simulink model "rl_forced_response"  (R2014b)
settings: Solver=ode45  StartTime=0.0  StopTime=1  RelTol=1e-3
libraries: powerlib x5
settings Model: Creator=Mashkoor Ahmed  LastModifiedBy=Mashkoor Ahmed

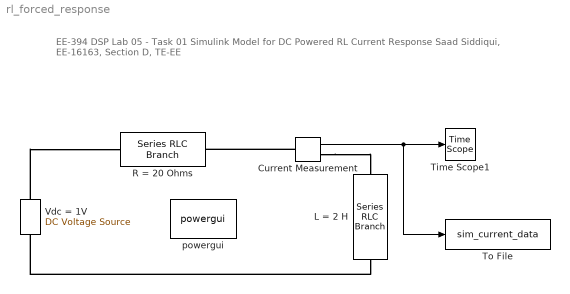
== system rl_forced_response ==
  note: EE-394 DSP Lab 05 - Task 01
      | Simulink Model for DC Powered RL Current Response
      | Saad Siddiqui, EE-16163, Section D, TE-EE
  Current Measurement : powerlib/Measurements/Current Measurement  PhasorSimulation=off  OutputType=Complex  PSBequivalent=0
  L = 2 H : powerlib/Elements/Series RLC Branch  LConnTagsString=__new0  RConnTagsString=__new0  BranchType=L  Resistance=1  Inductance=2  SetiL0=on  InitialCurrent=0  Capacitance=1e-6  Setx0=off  InitialVoltage=0  Measurements=None
  R = 20 Ohms : powerlib/Elements/Series RLC Branch  LConnTagsString=__new0  RConnTagsString=__new0  BranchType=R  Resistance=20  Inductance=0  SetiL0=off  InitialCurrent=0  Capacitance=1e-6  Setx0=off  InitialVoltage=0  Measurements=None
  Time Scope1 : TimeScope  DefaultConfigurationName=spbscopes.TimeScopeBlockCfg
  To File : ToFile  Filename=sim_current_data  MatrixName=simulink_current
  Vdc = 1V : powerlib/Electrical Sources/DC Voltage Source  Amplitude=1  Measurements=None
  powergui : powerlib/powergui  Priority=1  SimulationMode=Discrete  SolverType=Tustin/Backward Euler (TBE)  SampleTime=2e-2  frequency=60  SPID=off  DisableSnubberDevices=off  DisableRonSwitches=off  DisableVfSwitches=off  SwTol=0  DisplayEquations=off  Interpol=on  methode=off  Ts=100  frequencyindice=0  Pbase=100e6  ErrMax=1e-4  Iterations=50  UnitsV=kV  UnitsW=MW  FunctionMessages=off  echomessages=off  HookPort=off  EnableUseOfTLC=off  x0status=blocks  RestoreLinks=warning  ResistiveCurrentMeasurement=off  Frange=[0:2:500]  Ylog=off  Xlog=on  ShowGrid=off  save=off  variable=ZData  structure=0  ZoomFFT=off  StartTime=0.0  cycles=1  DisplayStyle=1  fundamental=60  FreqAxis=off  MaxFrequency=1000  frequencyindicesteady=1  RmsSteady=1  display=off
  wires:
  Current Measurement/1 -> To File/1, Time Scope1/1
  connections:
  Vdc = 1V/RConn1 -- R = 20 Ohms/LConn1
  Current Measurement/LConn1 -- R = 20 Ohms/RConn1
  Current Measurement/RConn1 -- L = 2 H/LConn1
  L = 2 H/RConn1 -- Vdc = 1V/LConn1
